simulink library "vmc"  (R2021b)
settings: Solver=VariableStepAuto  StartTime=0.0  StopTime=10.0  RelTol=1e-3
undefined symbols (not defined in the file): AVMC_ACCDeltaTqGradeGn_X_deg, AVMC_ACCDeltaTqIGain4OVRD_X_kph, AVMC_ACCDeltaTqIGain4OVRD_Y_mps2, AVMC_ACCDeltaTqIGain_X_kph, AVMC_ACCDeltaTqIGain_Y_mps2, AVMC_ACCDeltaTqPGain_X_kph, AVMC_ACCDeltaTqPGain_Y_kph, AVMC_ACCGradeofst_X_G, AVMC_ACCGradeofst_Y_pct, AVMC_ACCLoSpdTqLoLim4JP_X_kph, AVMC_ACCLoSpdTqLoLim4JP_Y_deg, AVMC_ACCLoSpdTqLowerLim_X_kph, AVMC_ACCLoSpdTqLowerLim_Y_deg, AVMC_ACCReqAccelGain_X_mps2, AVMC_ACCReqAccelGain_Y_enum, AVMC_ADSPosGFBDeltaTq_X_kph, AVMC_ADSPosGFBDeltaTq_Y_mps2, AVMC_AggressJerkPCT4AT_X_kph, AVMC_AggressJerkPCT_X_kph, AVMC_AggressLimitPCT4AT_X_kph, AVMC_AggressLimitPCT_X_kph, AVMC_DECGradeofst_X_G, AVMC_DECGradeofst_Y_pct, AVMC_DISCDeltaTqIGain_X_kph, AVMC_DISCDeltaTqIGain_Y_mps2, AVMC_DISCDeltaTqPGain_X_kph, AVMC_DISCDeltaTqPGain_Y_kph, AVMC_EPSForceSelect_X_enum, AVMC_EPSForceSelect_Y_enum, AVMC_EPSForceSelectD21_X_enum, AVMC_EPSForceSelectD21_Y_enum, AVMC_ESCRegenOut_X_kph, AVMC_ESCRegenOut_Y_Deg, AVMC_ESCRegenOutEnSpd_X_Deg, AVMC_EstPitchSlopeTs_X_kph, AVMC_GradeCompFlt_X_kph, AVMC_GyroYBandLo_X_Gps, AVMC_HoldResTq_X_kph, AVMC_ISOAccLimit_X_mps, AVMC_ISODecLimit_X_mps, AVMC_ISOJerk_X_mps, AVMC_LatESCRegenOut_X_kph, AVMC_LatESCRegenOut_Y_Deg, AVMC_LongAccDeadZone_X_kph, AVMC_LongAccFiltTsforP2_X_Gps, AVMC_MCPresBaseTq_X_bar, AVMC_MSAPedalOvrd_X_kph, AVMC_MSASpdBand_X_kph, AVMC_MSATqDownEndTq_X_kph, AVMC_MSATqDownTime_X_kph, AVMC_NegZCHoldTq_X_kph, AVMC_OPDDisSlideRate_X_Deg, AVMC_OVRD2ActSR2FCMCMD_X_mps2, AVMC_PedalTqRWhlRatio_X_Nm, AVMC_PedalTqRWhlRatio_Y_gps, AVMC_PedalTqRWhlSlipGain_X_rat, AVMC_PedalTqRWhlSlipGain_Y_kph, AVMC_PedalTqRWhSTRGGain_X_deg, AVMC_PedalTqRWhSTRGGain_Y_kph, AVMC_PosZCHoldTq_X_kph ... (+593)
libraries: hcu_lib x143, simulink x96, tqr x4, $bdroot x1, simulink_extras x1
(part 1 of 17)
settings Model: Creator=FVT22120  LastModifiedBy=lai17

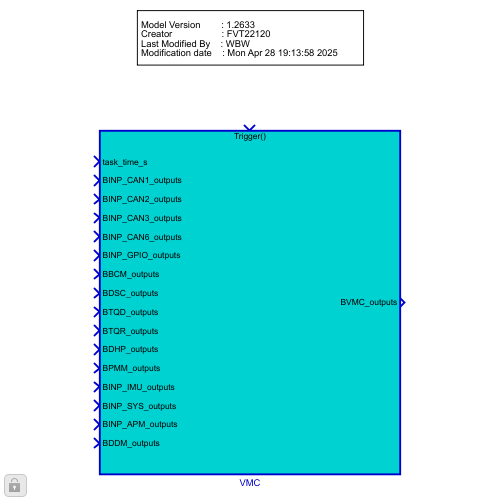
[thumbnail: Simulink's stored preview of the top-level diagram]
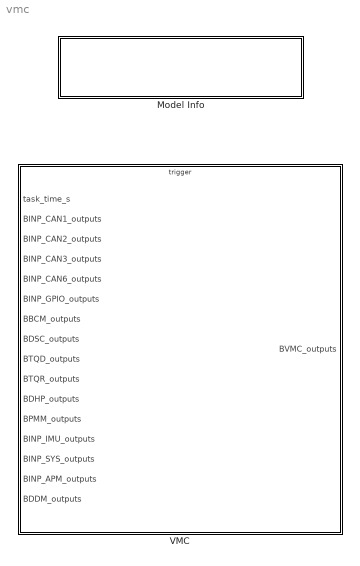
== system vmc ==
  Model Info : Subsystem  LoadFcn=slcm LoadBlock;  InitFcn=slcm('UpdateAllCMBlocksInThisModelInit')  mask(CMBlock){InitialSaveTempField=, InitialBlockCM=None, BlockCM=None, Frame=on, SaveTempField=, DisplayStringWithTags=|, MaskDisplayString=Model Version        : 1.2932\nCreator                   : FVT22120\nLast Modified By    : lai17\nModification date    : Wed Jul 23 21:49:31 2025, HorizontalTextAlignment=Left, LeftAlignmentValue=0.02, SourceBlockDiagram=tqr, TagMaxNumber=20, CMTag1=, CMTag2=, CMTag3=, CMTag4=, CMTag5=, CMTag6=, CMTag7=, CMTag8=, CMTag9=, CMTag10=, CMTag11=, CMTag12=, CMTag13=, CMTag14=, CMTag15=, CMTag16=, CMTag17=, CMTag18=, CMTag19=, CMTag20=}
      mask DisplayStringWithTags=|
      | Model Version        : %<ModelVersion>
      | Creator                   : %<Creator>
      | Last Modified By    : %<LastModifiedBy>
      | Modification date    : %<LastModificationDate>
      mask help: This block allows revision control information to be displayed within the model.
      settings: CopyFcn=slcm CopyBlock;  DeleteFcn=slcm Cancel;  PostSaveFcn=slcm('UpdateAllCMBlocksInThisModel')  NameChangeFcn=slcm Rename;  OpenFcn=slcm
      mask Display: text(str2num(LeftAlignmentValue), 0.5, MaskDisplayString, 'HorizontalAlignment', HorizontalTextAlignment)
  VMC : Subsystem
      settings: RTWSystemCode=Nonreusable function  RTWFcnNameOpts=Use subsystem name  RTWFileNameOpts=Use subsystem name

== system vmc/Model Info ==
  EmptySubsystem : Subsystem

== system vmc/VMC ==
  task_time_s : Inport
  BINP_CAN1_outputs : Inport  Port=2  OutDataTypeStr=Bus: BINP_CAN1_outputs
  BINP_CAN2_outputs : Inport  Port=3  OutDataTypeStr=Bus: BINP_CAN2_outputs
  BINP_CAN3_outputs : Inport  Port=4  OutDataTypeStr=Bus: BINP_CAN3_outputs
  BINP_CAN6_outputs : Inport  Port=5  OutDataTypeStr=Bus: BINP_CAN6_outputs
  BINP_GPIO_outputs : Inport  Port=6  OutDataTypeStr=Bus: BINP_GPIO_outputs
  BBCM_outputs : Inport  Port=7  OutDataTypeStr=Bus: BBCM_outputs
  BDSC_outputs : Inport  Port=8  OutDataTypeStr=Bus: BDSC_outputs
  BTQD_outputs : Inport  Port=9  OutDataTypeStr=Bus: BTQD_outputs
  BTQR_outputs : Inport  Port=10  OutDataTypeStr=Bus: BTQR_outputs
  BDHP_outputs : Inport  Port=11  OutDataTypeStr=Bus: BDHP_outputs
  BPMM_outputs : Inport  Port=12  OutDataTypeStr=Bus: BPMM_outputs
  BINP_IMU_outputs : Inport  Port=13  OutDataTypeStr=Bus: BINP_IMU_outputs
  BINP_SYS_outputs : Inport  Port=14  OutDataTypeStr=Bus: BINP_SYS_outputs
  BINP_APM_outputs : Inport  Port=15  OutDataTypeStr=Bus: BINP_APM_outputs
  BDDM_outputs : Inport  Port=16  OutDataTypeStr=Bus: BDDM_outputs
  Trigger : TriggerPort  TriggerType=function-call  VariantControl=(inherit)  PortDimensions=1
  Bus Creator2 : BusCreator  Inputs=160  OutDataTypeStr=Bus: BVMC_outputs  NonVirtualBus=on
  Bus Selector : BusSelector  OutputSignals=VINP_DriverSeatBeltCmd_flg,VINP_MeterIndVehSpeed_kph,VINP_BrkSwSta_flg,VINP_EPBSta_enum,VINP_ACCAvail_flg,VINP_AEBAvail_flg,VINP_ESCOFFStatus_enum,VINP_VehSpeed_kph,VINP_LFRawWhlSpeed_kph,VINP_LFRawWhlSpeedV_flg,VINP_RFRawWhlSpeed_kph,VINP_RFRawWhlSpeedV_flg,VINP_LRRawWhlSpeed_kph,VINP_LRRawWhlSpeedV_flg,VINP_RRRawWhlSpeed_kph,VINP_RRRawWhlSpeedV_flg,VINP_LatAccel_Gps,VINP_LatAccelV_flg,VINP_GRADE_Deg,VINP_LongAccel_Gps,VINP_MCPressure_bar,VINP_ESCADASSta_enum,VINP_FrRBCActive_flg,VINP_RrRBCActive_flg,VINP_FrntAxlTrqReqBrk_Nm,VINP_RearAxlTrqReqBrk_Nm,VINP_BrkPedalPos_pct,VINP_SASAngle_Deg,VINP_ESCActive_flg,VINP_YawRate_degps,VINP_RDCActive_enum,VINP_LFWhlRotDir_enum,VINP_LRWhlRotDir_enum,VINP_RFWhlRotDir_enum,VINP_RRWhlRotDir_enum,VINP_LongAccelV_flg
  Bus Selector1 : BusSelector  OutputSignals=VINP_DIDGetDynoMode_flg,VINP_VehicleType_enum,VINP_SWCType_enum
  Bus Selector10 : BusSelector  OutputSignals=VDHP_ActAPSPosn_pct
  Bus Selector11 : BusSelector  OutputSignals=VPMM_DrivetrainSelect_enum
  Bus Selector12 : BusSelector  OutputSignals=VINP_APSStaSystem_enum,VINP_APSDecReqA_flg,VINP_APSDecReq_mps2,VINP_APSReq_enum,VINP_APSShiftPosnReq_enum,VINP_APSSpeedCMD_kph,VINP_APSVMCReqA_flg,VINP_CAASVMCReqA_flg,VINP_APSVRqEPASCtrl_flg,VINP_APSRqEPASCtrl_flg,VINP_APSAngleTarget_Deg
  Bus Selector2 : BusSelector  OutputSignals=VBCM_DrDoorSW_flg
  Bus Selector3 : BusSelector  OutputSignals=VDDM_VCURAPSErrLv2_flg,VDDM_VCURAPSErrLv3_flg
  Bus Selector4 : BusSelector  OutputSignals=VTQD_DriverWhlTqDem_Nm,VTQD_CoordWhlTqDemFr_Nm,VTQD_CoordWhlTqDemRr_Nm,VTQD_GearActualPosn_enum,VTQD_ExternalTqAllow_flg,VTQD_LowIdleAccPedal_flg,VTQD_ExtShftAllow_flg,VTQD_FrEDUAvailBrkRgnTq_Nm,VTQD_RrEDUAvailBrkRgnTq_Nm,VTQD_APSStaSys_enum,VTQD_APSDecReqA_flg,VTQD_APSDecReq_mps2,VTQD_APSReq_enum,VTQD_AfterAvailableTqDemFr_Nm,VTQD_AfterAvailableTqDemRr_Nm,VTQD_EquivAccPedalSWSta_flg,VTQD_ExtDoorAllow_flg,VTQD_SpdCtrlSta_flg,VTQD_SpdCtrlMode_enum,VTQD_RegenMode_enum,VTQD_SetSpd_kph,VTQD_SWC2ResUpSta_flg,VTQD_SWC2SetdownSta_flg,VTQD_SWC2CancelSta_flg,VTQD_CreepBaseTqD_Nm,VTQD_VehActSpd_kph,VTQD_EVDriveMode_enum,VTQD_SWCCancelSta_flg,VTQD_SWCResUpSta_flg,VTQD_SWCSetdownSta_flg,VTQD_PreLoadPreEn_flg
  Bus Selector5 : BusSelector  OutputSignals=VINP_FrTMSpd_rpm,VINP_FrTMSpdNidec_rpm,VINP_RrTMSpd_rpm,VINP_RrTMSpdNidec_rpm,VINP_FrEDURealTMTq_Nm,VINP_FrEDURealTMTqNidec_Nm,VINP_FrEDURotateDirction_enum,VINP_FrEDURotateDirctionNidec_enum,VINP_RrEDURealTMTq_Nm,VINP_RrEDURealTMTqNidec_Nm,VINP_RrEDURotateDirction_enum,VINP_RrEDURotateDirctionNidec_enum
  Bus Selector6 : BusSelector  OutputSignals=VINP_BrakeSWGPIO_flg,VINP_HoodSW_flg
  Bus Selector7 : BusSelector  OutputSignals=VINP_ADASAEBSta_enum,VINP_ADASACCSta_enum,VINP_ACCRequiredAccel_mps2,VINP_ACCVehHoldReq_flg,VINP_ADASAEBReq_enum,VINP_ADASLKASta_enum,VINP_FCMLKAStrToqReq_Nm,VINP_FCMLKATOIFault_flg,VINP_FCMLKATOIAct_enum,VINP_ADASFaultSta_flg,VINP_AEBVehHoldReq_flg,VINP_ADASDBSReq_enum,VINP_ACCObjDist_m,VINP_ACCObjRelSpd_mps,VINP_TimeGapLevel_enum,VINP_HazardWarningReq_flg,VINP_ADASForceIdle_flg,VINP_RightTurnLightReq_flg,VINP_LeftTurnLightReq_flg,VINP_ForceLowBeam_enum,VINP_ACCJerkUpperLimit_mps3,VINP_ACCComfortBandUpper_mps2,VINP_ACCJerkLowerLimit_mps3,VINP_ACCComfortBandLower_mps2,VINP_ADASVehSpdLim_enum,VINP_ADASShftPosnReqA_flg,VINP_ADASShftPosnReq_enum,VINP_ADASFCWSta_enum,VINP_ADASLDWSta_enum,VINP_ADASFltWrnReq_flg,VINP_ACCObjDstLvl_enum,VINP_ACCTakeoverReq_flg,VINP_ADASWarningMsg_enum,VINP_ADASCAMSpdLim_enum,VINP_TargetType_enum,VINP_ADASSLIFSpdLim_enum,VINP_LKAHODDisplayWarning_flg,VINP_LKAHODSoundWarning_flg,VINP_ADASLFCSta_enum,VINP_ADASLaneModeL_enum,VINP_ADASLaneModeR_enum,VINP_ADASSLIFSta_enum,VINP_ADASISASta_enum,VINP_ADASLDWMute_flg,VINP_ADASFCWMute_flg,VINP_ADASLFCHandsOffWarning_enum,VINP_LVDADisabled_flg,VINP_LVDAMuteSta_enum,VINP_LVDAFailinfo_flg,VINP_LVDAWarning_flg,VINP_LVDAACCStatusInformation_flg,VINP_ADASLFCWarnSound_enum,VINP_FCMACCmode_enum,VINP_ADASLanetypeR_enum,VINP_ADASLanetypeL_enum,VINP_ADASLanecurveL_raw32,VINP_ADASLanecurveR_raw32,VINP_ADASDrvInputTqBoostAct_flg,VINP_ADASStrWhlAngCtrlStatus_flg,VINP_ADASMaxAngCtrlOutTqLimit_Nm,VINP_ADASDrvInputTqBoostGain_pct,VINP_ADASAngCtrlTqWeightGain_pct,VINP_ADASDesStrWhlAngCtrlCmd_Deg
  Bus Selector8 : BusSelector  OutputSignals=VINP_Distanceunit_flg,VINP_IVISWCVibModeSta_enum,VINP_SmartEcoModeSW_flg,VINP_IVIEPSForceCmd_enum
  Bus Selector9 : BusSelector  OutputSignals=VTQR_RrTMTqReq_Nm,VTQR_FrTMTqReq_Nm
  Constant : Constant  Value=ZERO_INT
  Constant1 : Constant  Value=ZERO_INT
  Constant{2..8,12..13} (9 alike) : Constant  Value=FALSE
  Ground{,1..9,14} (11 alike) : Ground
  Terminator : Terminator
  VMC : Subsystem
  BVMC_outputs : Outport  OutDataTypeStr=Bus:BVMC_outputs
  wires:
  Bus Selector/24 -> VMC/25(VINP_RrRBCActive_flg)  "<VINP_RrRBCActive_flg>"
  Bus Selector/23 -> VMC/24(VINP_FrRBCActive_flg)  "<VINP_FrRBCActive_flg>"
  BINP_CAN3_outputs/1 -> Bus Selector5/1
  Bus Selector/22 -> VMC/23(VINP_ESCADASSta_enum)  "<VINP_ESCADASSta_enum>"
  Bus Selector/21 -> VMC/22(VINP_MCPressure_bar)  "<VINP_MCPressure_bar>"
  Bus Selector7/9 -> VMC/65(VINP_LKATOIAct_enum)  "<VINP_FCMLKATOIAct_enum>"
  Bus Selector7/8 -> VMC/64(VINP_LKATOIFault_flg)  "<VINP_FCMLKATOIFault_flg>"
  Bus Selector8/1 -> VMC/38(VINP_Distanceunit_flg)  "<VINP_Distanceunit_flg>"
  Bus Selector/1 -> VMC/2(VINP_DriverSeatBeltCmd_flg)  "<VINP_DriverSeatBeltCmd_flg>"
  Bus Selector7/15 -> VMC/71(VINP_TimeGapLevel_enum)  "<VINP_TimeGapLevel_enum>"
  Bus Selector7/14 -> VMC/70(VINP_ACCObjRelSpd_mps)  "<VINP_ACCObjRelSpd_mps>"
  Bus Selector7/13 -> VMC/69(VINP_ACCObjDist_m)  "<VINP_ACCObjDist_m>"
  Bus Selector7/12 -> VMC/68(VINP_ADASDBSReq_enum)  "<VINP_ADASDBSReq_enum>"
  Bus Selector7/11 -> VMC/67(VINP_AEBVehHoldReq_flg)  "<VINP_AEBVehHoldReq_flg>"
  Bus Selector7/10 -> VMC/66(VINP_ADASFaultSta_flg)  "<VINP_ADASFaultSta_flg>"
  Bus Selector7/7 -> VMC/63(VINP_LKAStrToqReq_Nm)  "<VINP_FCMLKAStrToqReq_Nm>"
  Bus Selector7/6 -> VMC/62(VINP_ADASLKASta_enum)  "<VINP_ADASLKASta_enum>"
  Bus Selector7/5 -> VMC/61(VINP_ADASAEBReq_enum)  "<VINP_ADASAEBReq_enum>"
  Bus Selector7/4 -> VMC/60(VINP_ACCVehHoldReq_flg)  "<VINP_ACCVehHoldReq_flg>"
  Bus Selector7/3 -> VMC/59(VINP_ACCRequiredAccel_mps2)  "<VINP_ACCRequiredAccel_mps2>"
  Bus Selector7/2 -> VMC/58(VINP_ADASACCSta_enum)  "<VINP_ADASACCSta_enum>"
  Bus Selector7/1 -> VMC/57(VINP_ADASAEBSta_enum)  "<VINP_ADASAEBSta_enum>"
  BINP_CAN6_outputs/1 -> Bus Selector7/1
  Bus Selector6/1 -> VMC/120(VINP_BrakeSWGPIO_flg)  "<VINP_BrakeSWGPIO_flg>"
  BINP_GPIO_outputs/1 -> Bus Selector6/1
  task_time_s/1 -> VMC/1(task_time_s)
  Bus Selector/9 -> VMC/10(VINP_LFRawWhlSpeed_kph)  "<VINP_LFRawWhlSpeed_kph>"
  Bus Selector/10 -> VMC/11(VINP_LFRawWhlSpeedV_flg)  "<VINP_LFRawWhlSpeedV_flg>"
  Bus Selector/11 -> VMC/12(VINP_RFRawWhlSpeed_kph)  "<VINP_RFRawWhlSpeed_kph>"
  Bus Selector/12 -> VMC/13(VINP_RFRawWhlSpeedV_flg)  "<VINP_RFRawWhlSpeedV_flg>"
  Bus Selector/13 -> VMC/14(VINP_LRRawWhlSpeed_kph)  "<VINP_LRRawWhlSpeed_kph>"
  Bus Selector/14 -> VMC/15(VINP_LRRawWhlSpeedV_flg)  "<VINP_LRRawWhlSpeedV_flg>"
  Bus Selector/15 -> VMC/16(VINP_RRRawWhlSpeed_kph)  "<VINP_RRRawWhlSpeed_kph>"
  Bus Selector/16 -> VMC/17(VINP_RRRawWhlSpeedV_flg)  "<VINP_RRRawWhlSpeedV_flg>"
  Bus Selector/17 -> VMC/18(VINP_LatAccel_Gps)  "<VINP_LatAccel_Gps>"
  Bus Selector/6 -> VMC/7(VINP_AEBAvail_flg)  "<VINP_AEBAvail_flg>"
  Bus Selector/18 -> VMC/19(VINP_LatAccelV_flg)  "<VINP_LatAccelV_flg>"
  Bus Selector/5 -> VMC/6(VINP_ACCAvail_flg)  "<VINP_ACCAvail_flg>"
  Bus Selector/19 -> VMC/20(VINP_GRADE_Deg)  "<VINP_GRADE_Deg>"
  Bus Selector/2 -> VMC/3(VINP_MeterIndVehSpeed_kph)  "<VINP_MeterIndVehSpeed_kph>"
  Bus Selector/20 -> VMC/21(VINP_LongAccel_Gps)  "<VINP_LongAccel_Gps>"
  Bus Selector/7 -> VMC/8(VINP_ESCOFFStatus_enum)  "<VINP_ESCOFFStatus_enum>"
  Bus Selector/8 -> VMC/9(VINP_VehSpeed_kph)  "<VINP_VehSpeed_kph>"
  Bus Selector/4 -> VMC/5(VINP_EPBSta_enum)  "<VINP_EPBSta_enum>"
  Bus Selector/3 -> VMC/4(VINP_BrkSwSta_flg)  "<VINP_BrkSwSta_flg>"
  BTQD_outputs/1 -> Bus Selector4/1
  BDSC_outputs/1 -> Terminator/1
  Bus Selector2/1 -> VMC/138(VBCM_DrDoorSW_flg)  "<VBCM_DrDoorSW_flg>"
  BBCM_outputs/1 -> Bus Selector2/1
  BINP_CAN1_outputs/1 -> Bus Selector/1
  Bus Selector/25 -> VMC/26(VINP_FrntAxlTrqReqBrk_Nm)  "<VINP_FrntAxlTrqReqBrk_Nm>"
  Bus Selector/26 -> VMC/27(VINP_RearAxlTrqReqBrk_Nm)  "<VINP_RearAxlTrqReqBrk_Nm>"
  Bus Selector7/16 -> VMC/72(VINP_HazardWarningReq_flg)  "<VINP_HazardWarningReq_flg>"
  BTQR_outputs/1 -> Bus Selector9/1
  Bus Selector9/1 -> VMC/179(VTQR_RrTMTqReq_Nm)  "<VTQR_RrTMTqReq_Nm>"
  Bus Selector/27 -> VMC/28(VINP_BrkPedalPos_pct)  "<VINP_BrkPedalPos_pct>"
  BDHP_outputs/1 -> Bus Selector10/1
  Bus Selector10/1 -> VMC/181(VDHP_ActAPSPosn_pct)  "<VDHP_ActAPSPosn_pct>"
  VMC/1(VVMC_FeatSetSpdFinal_raw32) -> Bus Creator2/1
  VMC/2(VVMC_VehicleSpeed_mph) -> Bus Creator2/2
  VMC/3(VVMC_VehicleSpeed_kph) -> Bus Creator2/3
  VMC/4(VVMC_MeterIndSpeed_raw32) -> Bus Creator2/4
  VMC/5(VVMC_MeterIndSpeedForCalcu_kph) -> Bus Creator2/5
  VMC/6(VVMC_VMCAEBCtrlAvail_flg) -> Bus Creator2/6
  VMC/7(VVMC_VMCACCCtrlAvail_flg) -> Bus Creator2/7
  VMC/8(VVMC_VMCCCCtrlAvail_flg) -> Bus Creator2/8
  VMC/9(VVMC_VMCMSACtrlAvail_flg) -> Bus Creator2/9
  VMC/10(VVMC_FeatArbitrSta_enum) -> Bus Creator2/10
  VMC/11(VVMC_FeatReqSpd_kph) -> Bus Creator2/11
  VMC/12(VVMC_JerkPCT_pct) -> Bus Creator2/12
  VMC/13(VVMC_LimitPCT_pct) -> Bus Creator2/13
  VMC/14(VVMC_LFWhlSpeedRollAve_kph) -> Bus Creator2/14
  VMC/15(VVMC_RFWhlSpeedRollAve_kph) -> Bus Creator2/15
  VMC/16(VVMC_LRWhlSpeedRollAve_kph) -> Bus Creator2/16
  VMC/17(VVMC_RRWhlSpeedRollAve_kph) -> Bus Creator2/17
  VMC/18(VVMC_FrontRearSlipRatioCtrl_flg) -> Bus Creator2/18
  VMC/19(VVMC_RearWhlSlipRatioCtrl_flg) -> Bus Creator2/19
  VMC/20(VVMC_SingleWhlSlipRatioCtrl_flg) -> Bus Creator2/20
  VMC/21(VVMC_LatAccCtrl_flg) -> Bus Creator2/21
  VMC/22(VVMC_SafetyCtrl_flg) -> Bus Creator2/22
  VMC/23(VVMC_EstSlope_Deg) -> Bus Creator2/23
  VMC/24(VVMC_SPD2ACCAct_flg) -> Bus Creator2/24
  VMC/25(VVMC_AccCalcuPID_mps2) -> Bus Creator2/25
  VMC/26(VVMC_ISOAccLimit_mps2) -> Bus Creator2/26
  VMC/27(VVMC_ISODecLimit_mps2) -> Bus Creator2/27
  VMC/28(VVMC_ISOJerkLimit_mps3) -> Bus Creator2/28
  VMC/29(VVMC_ACCRequiredAccel_mps2) -> Bus Creator2/29
  VMC/30(VVMC_DISCReqAcc_mps2) -> Bus Creator2/30
  VMC/31(VVMC_FeatArbitrFinal_enum) -> Bus Creator2/31
  VMC/32(VVMC_ActACCRequiredAccel_mps2) -> Bus Creator2/32
  VMC/33(VVMC_LateralCtrl_flg) -> Bus Creator2/33
  VMC/34(VVMC_ADASLKASta_enum) -> Bus Creator2/34
  VMC/35(VVMC_LKAStrToqReq_Nm) -> Bus Creator2/35
  VMC/36(VVMC_LKATOIFault_flg) -> Bus Creator2/36
  VMC/37(VVMC_LKATOIAct_enum) -> Bus Creator2/37
  VMC/89(VVMC_ADASAEBSta_enum) -> Bus Creator2/89
  VMC/39(VVMC_ADASFaultSta_flg) -> Bus Creator2/39
  VMC/40(VVMC_AEBVehHoldReq_flg) -> Bus Creator2/40
  VMC/41(VVMC_ACCVehHoldReq_flg) -> Bus Creator2/41
  VMC/42(VVMC_ADASDBSReq_enum) -> Bus Creator2/42
  VMC/43(VVMC_ADASACCSta_enum) -> Bus Creator2/43
  VMC/44(VVMC_ACCObjDist_m) -> Bus Creator2/44
  VMC/45(VVMC_ACCObjRelSpd_mps) -> Bus Creator2/45
  VMC/46(VVMC_TimeGapLevel_enum) -> Bus Creator2/46
  VMC/47(VVMC_ACCJerkUpperLimit_mps3) -> Bus Creator2/47
  VMC/48(VVMC_ACCComfortBandUpper_mps2) -> Bus Creator2/48
  VMC/49(VVMC_ACCJerkLowerLimit_mps3) -> Bus Creator2/49
  VMC/50(VVMC_ACCComfortBandLower_mps2) -> Bus Creator2/50
  VMC/51(VVMC_ADASVehSpdLim_raw32) -> Bus Creator2/51
  VMC/52(VVMC_ADASShftPosnReqA_flg) -> Bus Creator2/52
  VMC/53(VVMC_ADASShftPosnReq_enum) -> Bus Creator2/53
  VMC/54(VVMC_ADASForceIdle_flg) -> Bus Creator2/54
  VMC/55(VVMC_HazardWarningReq_flg) -> Bus Creator2/55
  VMC/56(VVMC_RightTurnLightReq_flg) -> Bus Creator2/56
  VMC/57(VVMC_LeftTurnLightReq_flg) -> Bus Creator2/57
  VMC/58(VVMC_ADASFCWSta_enum) -> Bus Creator2/58
  VMC/59(VVMC_ADASLDWSta_enum) -> Bus Creator2/59
  VMC/60(VVMC_ADASFltWrnReq_flg) -> Bus Creator2/60
  VMC/61(VVMC_ACCObjDstLvl_enum) -> Bus Creator2/61
  VMC/62(VVMC_ForceLowBeam_enum) -> Bus Creator2/62
  VMC/63(VVMC_ACCTakeoverReq_flg) -> Bus Creator2/63
  VMC/64(VVMC_ADASWarningMsg_enum) -> Bus Creator2/64
  VMC/65(VVMC_ADASCAMSpdLim_enum) -> Bus Creator2/65
  VMC/66(VVMC_TargetType_enum) -> Bus Creator2/66
  VMC/67(VVMC_ADASSLIFSpdLim_enum) -> Bus Creator2/67
  VMC/68(VVMC_LKAHODDisplayWarning_flg) -> Bus Creator2/68
  VMC/69(VVMC_LKAHODSoundWarning_flg) -> Bus Creator2/69
  VMC/70(VVMC_ADASLFCSta_enum) -> Bus Creator2/70
  VMC/71(VVMC_ADASLaneModeL_enum) -> Bus Creator2/71
  VMC/72(VVMC_ADASLaneModeR_enum) -> Bus Creator2/72
  VMC/73(VVMC_ADASSLIFSta_enum) -> Bus Creator2/73
  VMC/74(VVMC_ADASISASta_enum) -> Bus Creator2/74
  VMC/75(VVMC_ADASLDWMute_flg) -> Bus Creator2/75
  VMC/76(VVMC_ADASFCWMute_flg) -> Bus Creator2/76
  VMC/77(VVMC_ADASLFCHandsOffWarning_enum) -> Bus Creator2/77
  VMC/78(VVMC_LVDADisabled_flg) -> Bus Creator2/78
  VMC/79(VVMC_LVDAMuteSta_enum) -> Bus Creator2/79
  VMC/80(VVMC_LVDAFailinfo_flg) -> Bus Creator2/80
  VMC/81(VVMC_LVDAWarning_flg) -> Bus Creator2/81
  VMC/82(VVMC_LVDAACCStatusInformation_flg) -> Bus Creator2/82
  VMC/83(VVMC_ADASLFCWarnSound_enum) -> Bus Creator2/83
  VMC/84(VVMC_FCMACCmode_enum) -> Bus Creator2/84
  VMC/85(VVMC_ADASLanetypeR_enum) -> Bus Creator2/85
  VMC/86(VVMC_ADASLanetypeL_enum) -> Bus Creator2/86
  VMC/87(VVMC_ADASLanecurveL_raw32) -> Bus Creator2/87
  VMC/88(VVMC_ADASLanecurveR_raw32) -> Bus Creator2/88
  VMC/38(VVMC_ADASAEBReq_enum) -> Bus Creator2/38
  VMC/90(VVMC_FCMLDWRequest_enum) -> Bus Creator2/90
  VMC/91(VVMC_FCMLDWFault_flg) -> Bus Creator2/91
  VMC/92(VVMC_ADASActive_flg) -> Bus Creator2/92
  VMC/93(VVMC_ACCCtrlAvail_flg) -> Bus Creator2/93
  VMC/94(VVMC_ADASNegReq_flg) -> Bus Creator2/94
  VMC/95(VVMC_ACCPedalOvrd_flg) -> Bus Creator2/95
  VMC/96(VVMC_ADASWhlTqReq_Nm) -> Bus Creator2/96
  VMC/97(VVMC_AccPedalOvrdDISC_flg) -> Bus Creator2/97
  VMC/98(VVMC_RearTqRatio_rat) -> Bus Creator2/98
  VMC/99(VVMC_TimeGapCalcu_s) -> Bus Creator2/99
  VMC/100(VVMC_CCCtrlSta_enum) -> Bus Creator2/100
  VMC/101(VVMC_CruzActive_flg) -> Bus Creator2/101
  VMC/102(VVMC_CCPedalOvrd_flg) -> Bus Creator2/102
  VMC/103(VVMC_CruzWhlTqReq_Nm) -> Bus Creator2/103
  VMC/104(VVMC_MSACtrlSta_enum) -> Bus Creator2/104
  VMC/105(VVMC_MSAActive_flg) -> Bus Creator2/105
  VMC/106(VVMC_MSAWhlTqReq_Nm) -> Bus Creator2/106
  VMC/107(VVMC_APSCtrlAvail_flg) -> Bus Creator2/107
  VMC/108(VVMC_APSActive_flg) -> Bus Creator2/108
  VMC/109(VVMC_APSSpeedCMD_kph) -> Bus Creator2/109
  VMC/110(VVMC_APSShiftPosnReq_enum) -> Bus Creator2/110
  VMC/111(VVMC_APSStaSys_enum) -> Bus Creator2/111
  VMC/112(VVMC_APSDecReqA_flg) -> Bus Creator2/112
  VMC/113(VVMC_APSDecReq_mps2) -> Bus Creator2/113
  VMC/114(VVMC_APSReq_enum) -> Bus Creator2/114
  VMC/115(VVMC_LongAcc_Gps) -> Bus Creator2/115
  VMC/116(VVMC_RawWhlSpdSlideRate_pct) -> Bus Creator2/116
  VMC/117(VVMC_LFWhlSpdSlideRate_pct) -> Bus Creator2/117
  VMC/118(VVMC_RFWhlSpdSlideRate_pct) -> Bus Creator2/118
  VMC/119(VVMC_LRWhlSpdSlideRate_pct) -> Bus Creator2/119
  VMC/120(VVMC_RRWhlSpdSlideRate_pct) -> Bus Creator2/120
  VMC/121(VVMC_PredictVehSpd_kph) -> Bus Creator2/121
  VMC/122(VVMC_LF4WhlSpdSlideRate_pct) -> Bus Creator2/122
  VMC/123(VVMC_RF4WhlSpdSlideRate_pct) -> Bus Creator2/123
  VMC/124(VVMC_LR4WhlSpdSlideRate_pct) -> Bus Creator2/124
  VMC/125(VVMC_RR4WhlSpdSlideRate_pct) -> Bus Creator2/125
  VMC/126(VVMC_4WhlSpdSlideRate_pct) -> Bus Creator2/126
  VMC/127(VVMC_ActMaxSlideRate_pct) -> Bus Creator2/127
  VMC/128(VVMC_ActLFSlideRate_pct) -> Bus Creator2/128
  VMC/129(VVMC_ActRFSlideRate_pct) -> Bus Creator2/129
  VMC/130(VVMC_ActLRSlideRate_pct) -> Bus Creator2/130
  VMC/131(VVMC_ActRRSlideRate_pct) -> Bus Creator2/131
  VMC/132(VVMC_AltLWhlSlideRate_pct) -> Bus Creator2/132
  VMC/133(VVMC_AltRWhlSlideRate_pct) -> Bus Creator2/133
  VMC/134(VVMC_AltWhlSlideRate_pct) -> Bus Creator2/134
  VMC/135(VVMC_CCMSASpdWar_flg) -> Bus Creator2/135
  Bus Selector9/2 -> VMC/180(VTQR_FrTMTqReq_Nm)  "<VTQR_FrTMTqReq_Nm>"
  Bus Selector7/20 -> VMC/76(VINP_ForceLowBeam_enum)  "<VINP_ForceLowBeam_enum>"
  Bus Selector7/18 -> VMC/74(VINP_RightTurnLightReq_flg)  "<VINP_RightTurnLightReq_flg>"
  Bus Selector7/19 -> VMC/75(VINP_LeftTurnLightReq_flg)  "<VINP_LeftTurnLightReq_flg>"
  Bus Selector7/17 -> VMC/73(VINP_ADASForceIdle_flg)  "<VINP_ADASForceIdle_flg>"
  BINP_CAN2_outputs/1 -> Bus Selector8/1
  Bus Selector7/21 -> VMC/77(VINP_ACCJerkUpperLimit_mps3)  "<VINP_ACCJerkUpperLimit_mps3>"
  Bus Selector7/22 -> VMC/78(VINP_ACCComfortBandUpper_mps2)  "<VINP_ACCComfortBandUpper_mps2>"
  Bus Selector7/23 -> VMC/79(VINP_ACCJerkLowerLimit_mps3)  "<VINP_ACCJerkLowerLimit_mps3>"
  Bus Selector7/24 -> VMC/80(VINP_ACCComfortBandLower_mps2)  "<VINP_ACCComfortBandLower_mps2>"
  Bus Selector7/25 -> VMC/81(VINP_ADASVehSpdLim_raw32)  "<VINP_ADASVehSpdLim_enum>"
  Bus Selector7/26 -> VMC/82(VINP_ADASShftPosnReqA_flg)  "<VINP_ADASShftPosnReqA_flg>"
  Bus Selector7/27 -> VMC/83(VINP_ADASShftPosnReq_enum)  "<VINP_ADASShftPosnReq_enum>"
  Bus Selector7/28 -> VMC/84(VINP_ADASFCWSta_enum)  "<VINP_ADASFCWSta_enum>"
  Bus Selector7/29 -> VMC/85(VINP_ADASLDWSta_enum)  "<VINP_ADASLDWSta_enum>"
  Bus Selector7/30 -> VMC/86(VINP_ADASFltWrnReq_flg)  "<VINP_ADASFltWrnReq_flg>"
  Bus Selector7/31 -> VMC/87(VINP_ACCObjDstLvl_enum)  "<VINP_ACCObjDstLvl_enum>"
  Bus Selector7/32 -> VMC/88(VINP_ACCTakeoverReq_flg)  "<VINP_ACCTakeoverReq_flg>"
  Bus Selector7/33 -> VMC/89(VINP_ADASWarningMsg_enum)  "<VINP_ADASWarningMsg_enum>"
  Bus Selector7/34 -> VMC/90(VINP_ADASCAMSpdLim_enum)  "<VINP_ADASCAMSpdLim_enum>"
  Bus Selector7/35 -> VMC/91(VINP_TargetType_enum)  "<VINP_TargetType_enum>"
  Bus Selector7/36 -> VMC/92(VINP_ADASSLIFSpdLim_enum)  "<VINP_ADASSLIFSpdLim_enum>"
  Bus Selector7/37 -> VMC/93(VINP_LKAHODDisplayWarning_flg)  "<VINP_LKAHODDisplayWarning_flg>"
  Bus Selector7/38 -> VMC/94(VINP_LKAHODSoundWarning_flg)  "<VINP_LKAHODSoundWarning_flg>"
  Bus Selector7/39 -> VMC/95(VINP_ADASLFCSta_enum)  "<VINP_ADASLFCSta_enum>"
  Bus Selector7/40 -> VMC/96(VINP_ADASLaneModeL_enum)  "<VINP_ADASLaneModeL_enum>"
  Bus Selector7/41 -> VMC/97(VINP_ADASLaneModeR_enum)  "<VINP_ADASLaneModeR_enum>"
  Bus Selector7/42 -> VMC/98(VINP_ADASSLIFSta_enum)  "<VINP_ADASSLIFSta_enum>"
  Bus Selector7/43 -> VMC/99(VINP_ADASISASta_enum)  "<VINP_ADASISASta_enum>"
  Bus Selector7/44 -> VMC/100(VINP_ADASLDWMute_flg)  "<VINP_ADASLDWMute_flg>"
  Bus Selector7/45 -> VMC/101(VINP_ADASFCWMute_flg)  "<VINP_ADASFCWMute_flg>"
  Bus Selector7/46 -> VMC/102(VINP_ADASLFCHandsOffWarning_enum)  "<VINP_ADASLFCHandsOffWarning_enum>"
  Bus Selector7/47 -> VMC/103(VINP_LVDADisabled_flg)  "<VINP_LVDADisabled_flg>"
  Bus Selector7/48 -> VMC/104(VINP_LVDAMuteSta_enum)  "<VINP_LVDAMuteSta_enum>"
  Bus Selector7/49 -> VMC/105(VINP_LVDAFailinfo_flg)  "<VINP_LVDAFailinfo_flg>"
  Bus Selector7/50 -> VMC/106(VINP_LVDAWarning_flg)  "<VINP_LVDAWarning_flg>"
  Bus Selector7/51 -> VMC/107(VINP_LVDAACCStatusInformation_flg)  "<VINP_LVDAACCStatusInformation_flg>"
  Bus Selector7/52 -> VMC/108(VINP_ADASLFCWarnSound_enum)  "<VINP_ADASLFCWarnSound_enum>"
  Bus Selector/28 -> VMC/29(VINP_SASAngle_Deg)  "<VINP_SASAngle_Deg>"
  BPMM_outputs/1 -> Bus Selector11/1
  Bus Selector11/1 -> VMC/182(<VPMM_DrivetrainSelect_enum>)  "<VPMM_DrivetrainSelect_enum>"
  VMC/136(VVMC_IMUEnaCmd_flg) -> Bus Creator2/136
  VMC/137(VVMC_RWDRDCActive_enum) -> Bus Creator2/137
  Bus Selector/29 -> VMC/30(VINP_ESCActive_flg)  "<VINP_ESCActive_flg>"
  Bus Selector/30 -> VMC/31(VINP_YawRate_degps)  "<VINP_YawRate_degps>"
  Bus Selector/31 -> VMC/32(VINP_RDCActive_enum)  "<VINP_RDCActive_enum>"
  VMC/138(VVMC_MSAWhlTqActive_flg) -> Bus Creator2/138
  Bus Selector/32 -> VMC/33(VINP_LFWhlRotDir_enum)  "<VINP_LFWhlRotDir_enum>"
  Bus Selector/33 -> VMC/34(VINP_LRWhlRotDir_enum)  "<VINP_LRWhlRotDir_enum>"
  Bus Selector/34 -> VMC/35(VINP_RFWhlRotDir_enum)  "<VINP_RFWhlRotDir_enum>"
  Bus Selector/35 -> VMC/36(VINP_RRWhlRotDir_enum)  "<VINP_RRWhlRotDir_enum>"
  BINP_IMU_outputs/1 -> VMC/183(BINP_IMU_outputs)
  VMC/139(VVMC_RDCEnSlideRate_pct) -> Bus Creator2/139
  VMC/140(VVMC_ActStESCYaw_Dps) -> Bus Creator2/140
  Bus Selector6/2 -> VMC/121(VINP_HoodSW_flg)  "<VINP_HoodSW_flg>"
  BINP_APM_outputs/1 -> Bus Selector12/1
  VMC/141(VVMC_ACCOvrdMemTq_Nm) -> Bus Creator2/141
  Bus Selector12/1 -> VMC/127(VINP_APSStaSystem_enum)  "<VINP_APSStaSystem_enum>"
  Ground3/1 -> VMC/122(APP_SpdLimit_flg)
  Ground14/1 -> VMC/123(APP_SpdLimit)
  Bus Selector7/57 -> VMC/113(VINP_ADASLanecurveR_raw32)  "<VINP_ADASLanecurveR_raw32>"
  Bus Selector7/55 -> VMC/111(VINP_ADASLanetypeL_enum)  "<VINP_ADASLanetypeL_enum>"
  Bus Selector7/56 -> VMC/112(VINP_ADASLanecurveL_raw32)  "<VINP_ADASLanecurveL_raw32>"
  Bus Selector7/54 -> VMC/110(VINP_ADASLanetypeR_enum)  "<VINP_ADASLanetypeR_enum>"
  Bus Selector7/53 -> VMC/109(VINP_FCMACCmode_enum)  "<VINP_FCMACCmode_enum>"
  VMC/142(VVMC_CAASCtrlAvail_flg) -> Bus Creator2/142
  VMC/143(VVMC_CAASActive_flg) -> Bus Creator2/143
  VMC/144("VVMC_ExtraMSACtrlSta_enum ") -> Bus Creator2/144
  VMC/145(VVMC_CalibratedAccX_G) -> Bus Creator2/145
  VMC/146(VVMC_CalibratedAccY_G) -> Bus Creator2/146
  VMC/147(VVMC_CalibratedAccZ_G) -> Bus Creator2/147
  VMC/148(VVMC_CalibratedGyroX_Dps) -> Bus Creator2/148
  VMC/149(VVMC_CalibratedGyroY_Dps) -> Bus Creator2/149
  VMC/150(VVMC_CalibratedGyroZ_Dps) -> Bus Creator2/150
  Bus Selector8/2 -> VMC/39(VINP_IVISWCVibModeSta_enum)  "<VINP_IVISWCVibModeSta_enum>"
  VMC/151(VVMC_SetACCDisableAPS_flg) -> Bus Creator2/151
  Bus Selector8/3 -> VMC/40(VINP_SmartEcoModeSW_flg)  "<VINP_SmartEcoModeSW_flg>"
  Bus Selector12/2 -> VMC/128(VINP_APSDecReqA_flg)  "<VINP_APSDecReqA_flg>"
  Bus Selector12/3 -> VMC/129(VINP_APSDecReq_mps2)  "<VINP_APSDecReq_mps2>"
  Bus Selector12/4 -> VMC/130(VINP_APSReq_enum)  "<VINP_APSReq_enum>"
  Bus Selector12/5 -> VMC/131(VINP_APSShiftPosnReq_enum)  "<VINP_APSShiftPosnReq_enum>"
  Bus Selector12/6 -> VMC/132(VINP_APSSpeedCMD_kph)  "<VINP_APSSpeedCMD_kph>"
  Bus Selector12/7 -> VMC/133(VINP_APSVMCReqA_flg)  "<VINP_APSVMCReqA_flg>"
  Bus Selector12/8 -> VMC/134(VINP_CAASVMCReqA_flg)  "<VINP_CAASVMCReqA_flg>"
  BINP_SYS_outputs/1 -> Bus Selector1/1
  Bus Selector1/1 -> VMC/124(VINP_DIDGetDynoMode_flg)  "<VINP_DIDGetDynoMode_flg>"
  Ground/1 -> VMC/139(VDSC_DISCTurn_flg)
  Ground1/1 -> VMC/140(VDSC_DISCSta_enum)
  Ground2/1 -> VMC/141(VDSC_DISCTargetSpd_kph)
  Ground5/1 -> VMC/142(VDSC_TurningSpdMovingflat_kph)
  Ground6/1 -> VMC/143(VDSC_AutoTurnMode_flg)
  Ground7/1 -> VMC/144(VDSC_AccDecResp_flg)
  Ground8/1 -> VMC/145(VDSC_PreACC_flg)
  Ground9/1 -> VMC/146(VDSC_PreACC_mps2)
  Bus Selector5/4 -> VMC/48(VINP_RrTMSpdNidec_rpm)  "<VINP_RrTMSpdNidec_rpm>"
  Bus Selector5/2 -> VMC/46(VINP_FrTMSpdNidec_rpm)  "<VINP_FrTMSpdNidec_rpm>"
  Bus Selector5/1 -> VMC/45(VINP_FrTMSpd_rpm)  "<VINP_FrTMSpd_rpm>"
  Bus Selector5/3 -> VMC/47(VINP_RrTMSpd_rpm)  "<VINP_RrTMSpd_rpm>"
  Bus Selector7/63 -> VMC/119(VINP_ADASDesStrWhlAngCtrlCmd_Deg)  "<VINP_ADASDesStrWhlAngCtrlCmd_Deg>"
  Bus Selector7/62 -> VMC/118(VINP_ADASAngCtrlTqWeightGain_pct)  "<VINP_ADASAngCtrlTqWeightGain_pct>"
  Bus Selector7/61 -> VMC/117(VINP_ADASDrvInputTqBoostGain_pct)  "<VINP_ADASDrvInputTqBoostGain_pct>"
  Bus Selector7/60 -> VMC/116(VINP_ADASMaxAngCtrlOutTqLimit_Nm)  "<VINP_ADASMaxAngCtrlOutTqLimit_Nm>"
  Bus Selector7/58 -> VMC/114(VINP_ADASDrvInputTqBoostAct_flg)  "<VINP_ADASDrvInputTqBoostAct_flg>"
  VMC/152(VVMC_FDCVMCAPSVRqEPSCtrl_flg) -> Bus Creator2/152
  VMC/153(VVMC_FDCVMCAPSAngleTarget_deg) -> Bus Creator2/153
  VMC/154(VVMC_FDCVMCAPSRqEPSCtrl_flg) -> Bus Creator2/154
  Bus Selector12/9 -> VMC/135(VINP_APSVRqEPASCtrl_flg)  "<VINP_APSVRqEPASCtrl_flg>"
  Bus Selector12/10 -> VMC/136(VINP_APSRqEPASCtrl_flg)  "<VINP_APSRqEPASCtrl_flg>"
  Bus Selector12/11 -> VMC/137(VINP_APSAngleTarget_Deg)  "<VINP_APSAngleTarget_Deg>"
  VMC/155(VVMC_FDCVMCAngCtrlTqWtGn_pct) -> Bus Creator2/155
  VMC/156(VVMC_FDCVMCDrInpTqBstAct_flg) -> Bus Creator2/156
  VMC/157(VVMC_FDCVMCMaxAngCtrlOutTqLim_Nm) -> Bus Creator2/157
  VMC/158(VVMC_FDCVMCDrInpTqBstGn_pct) -> Bus Creator2/158
  Bus Creator2/1 -> BVMC_outputs/1  "BVMC_outputs"
  Constant2/1 -> VMC/184(VDDM_VMCLongCtrlProhibited_flg)
  Constant5/1 -> VMC/187(VDDM_ESC5Err_flg)
  Constant4/1 -> VMC/186(VDDM_ESC1Err_flg)
  Constant3/1 -> VMC/185(VDDM_VMCLatCtrlProhibited_flg)
  BDDM_outputs/1 -> Bus Selector3/1
  Constant6/1 -> VMC/188(VDDM_VMCEPSErr_flg)
  Bus Selector7/59 -> VMC/115(VINP_ADASStrWhlAngCtrlStatus_flg)  "<VINP_ADASStrWhlAngCtrlStatus_flg>"
  Bus Selector3/1 -> VMC/189(VDDM_VCURAPSErrLv2_flg)  "<VDDM_VCURAPSErrLv2_flg>"
  Bus Selector3/2 -> VMC/190(VDDM_VCURAPSErrLv3_flg)  "<VDDM_VCURAPSErrLv3_flg>"
  Ground4/1 -> VMC/193(VINP_SCPSystemMode_enum)
  Bus Selector4/1 -> VMC/147(VTQD_DriverWhlTqDem_Nm)  "<VTQD_DriverWhlTqDem_Nm>"
  Bus Selector4/2 -> VMC/148(VTQD_CoordWhlTqDemFr_Nm)  "<VTQD_CoordWhlTqDemFr_Nm>"
  Bus Selector4/3 -> VMC/149(VTQD_CoordWhlTqDemRr_Nm)  "<VTQD_CoordWhlTqDemRr_Nm>"
  Bus Selector4/4 -> VMC/150(VTQD_GearActualPosn_enum)  "<VTQD_GearActualPosn_enum>"
  Bus Selector4/5 -> VMC/151(VTQD_ExternalTqAllow_flg)  "<VTQD_ExternalTqAllow_flg>"
  Bus Selector4/6 -> VMC/152(VTQD_LowIdleAccPedal_flg)  "<VTQD_LowIdleAccPedal_flg>"
  Bus Selector4/7 -> VMC/153(VTQD_ExtShftAllow_flg)  "<VTQD_ExtShftAllow_flg>"
  Bus Selector4/8 -> VMC/154(VTQD_FrEDUAvailBrkRgnTq_Nm)  "<VTQD_FrEDUAvailBrkRgnTq_Nm>"
  Bus Selector4/9 -> VMC/155(VTQD_RrEDUAvailBrkRgnTq_Nm)  "<VTQD_RrEDUAvailBrkRgnTq_Nm>"
  Bus Selector4/10 -> VMC/156(VTQD_APSStaSys_enum)  "<VTQD_APSStaSys_enum>"
  Bus Selector4/11 -> VMC/157(VTQD_APSDecReqA_flg)  "<VTQD_APSDecReqA_flg>"
  Bus Selector4/12 -> VMC/158(VTQD_APSDecReq_mps2)  "<VTQD_APSDecReq_mps2>"
  Bus Selector4/13 -> VMC/159(VTQD_APSReq_enum)  "<VTQD_APSReq_enum>"
  Bus Selector4/14 -> VMC/160(VTQD_AfterAvailableTqDemFr_Nm)  "<VTQD_AfterAvailableTqDemFr_Nm>"
  Bus Selector4/15 -> VMC/161(VTQD_AfterAvailableTqDemRr_Nm)  "<VTQD_AfterAvailableTqDemRr_Nm>"
  Bus Selector4/16 -> VMC/162(VTQD_EquivAccPedalSWSta_flg)  "<VTQD_EquivAccPedalSWSta_flg>"
  Bus Selector4/30 -> VMC/176(VTQD_SWC1SetdownSta_flg)  "<VTQD_SWCSetdownSta_flg>"
  Bus Selector4/29 -> VMC/175(VTQD_SWC1ResUpSta_flg)  "<VTQD_SWCResUpSta_flg>"
  Bus Selector4/28 -> VMC/174(VTQD_SWC1CANCELSta_flg)  "<VTQD_SWCCancelSta_flg>"
  Bus Selector4/27 -> VMC/173(VTQD_EVDriveMode_enum)  "<VTQD_EVDriveMode_enum>"
  Bus Selector4/26 -> VMC/172(VTQD_VehActSpd_kph)  "<VTQD_VehActSpd_kph>"
  Bus Selector4/25 -> VMC/171(VTQD_CreepBaseTqD_Nm)  "<VTQD_CreepBaseTqD_Nm>"
  Bus Selector4/24 -> VMC/170(VTQD_SWC2CANCELSta_flg)  "<VTQD_SWC2CancelSta_flg>"
  Bus Selector4/23 -> VMC/169(VTQD_SWC2SetdownSta_flg)  "<VTQD_SWC2SetdownSta_flg>"
  Bus Selector4/22 -> VMC/168(VTQD_SWC2ResUpSta_flg)  "<VTQD_SWC2ResUpSta_flg>"
  Bus Selector4/21 -> VMC/167(VTQD_SetSpd_kph)  "<VTQD_SetSpd_kph>"
  Bus Selector4/20 -> VMC/166(VTQD_RegenMode_enum)  "<VTQD_RegenMode_enum>"
  Bus Selector4/19 -> VMC/165(VTQD_SpdCtrlMode_enum)  "<VTQD_SpdCtrlMode_enum>"
  Bus Selector4/18 -> VMC/164(VTQD_SpdCtrlSta_flg)  "<VTQD_SpdCtrlSta_flg>"
  Bus Selector4/17 -> VMC/163(VTQD_ExtDoorAllow_flg)  "<VTQD_ExtDoorAllow_flg>"
  Bus Selector1/2 -> VMC/125(VINP_VehicleType_enum)  "<VINP_VehicleType_enum>"
  Bus Selector1/3 -> VMC/126(VINP_SWCType_enum)  "<VINP_SWCType_enum>"
  Constant13/1 -> VMC/191(VDDM_LimpHomeAct_flg)
  Constant12/1 -> VMC/192(VDDM_VCUMSAErr_flg)
  VMC/160(VVMC_DMSModeCmd_enum) -> Bus Creator2/160
  Constant8/1 -> VMC/178(VTQD_EPBCarWashMode_flg)
  Bus Selector8/4 -> VMC/41(VINP_IVIEPSForceCmd_enum)  "<VINP_IVIEPSForceCmd_enum>"
  VMC/159(VVMC_VehPitchAngleSta_enum) -> Bus Creator2/159
  Bus Selector5/5 -> VMC/49(VINP_FrEDURealTMTq_Nm)  "<VINP_FrEDURealTMTq_Nm>"
  Bus Selector5/6 -> VMC/50(VINP_FrEDURealTMTqNidec_Nm)  "<VINP_FrEDURealTMTqNidec_Nm>"
  Bus Selector5/9 -> VMC/53(VINP_RrEDURealTMTq_Nm)  "<VINP_RrEDURealTMTq_Nm>"
  Bus Selector5/10 -> VMC/54(VINP_RrEDURealTMTqNidec_Nm)  "<VINP_RrEDURealTMTqNidec_Nm>"
  Bus Selector5/7 -> VMC/51(VINP_FrEDURotateDirction_enum)  "<VINP_FrEDURotateDirction_enum>"
  Bus Selector5/8 -> VMC/52(VINP_FrEDURotateDirctionNidec_enum)  "<VINP_FrEDURotateDirctionNidec_enum>"
  Bus Selector5/11 -> VMC/55(VINP_RrEDURotateDirction_enum)  "<VINP_RrEDURotateDirction_enum>"
  Bus Selector5/12 -> VMC/56(VINP_RrEDURotateDirctionNidec_enum)  "<VINP_RrEDURotateDirctionNidec_enum>"
  Bus Selector/36 -> VMC/37(VINP_LongAccelV_flg)  "<VINP_LongAccelV_flg>"
  Bus Selector4/31 -> VMC/177(VTQD_PreLoadPreEn_flg)  "<VTQD_PreLoadPreEn_flg>"
  Constant/1 -> VMC/42(VINP_DMSStatus_enum)
  Constant1/1 -> VMC/43(VINP_DMSWarningFatigue_enum)
  Constant7/1 -> VMC/44(VINP_DMSWarningUnresponsive_flg)

== system vmc/Model Info/EmptySubsystem ==
